simulink model "cl_cm"  (R2021b)
settings: Solver=VariableStepAuto  StartTime=0.0  StopTime=5  RelTol=1e-3
values from neighbouring files (symbols this model uses):
  cl0 = 0.26318895    [model_main.m]
  cla = 5.5497917    [model_main.m]
  clad = 0.008081279    [model_main.m]
  cm0 = 0.08960583    [model_main.m]
  cma = -0.26464918    [model_main.m]
  cmad = -0.018147167    [model_main.m]
  U = 40.00    (= 40)    [model_main.m]
settings Model: Creator=stevenfang  LastModifiedBy=stevenfang

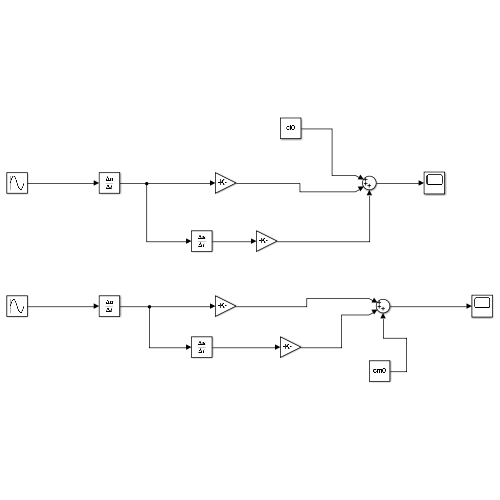
[thumbnail: Simulink's stored preview of the top-level diagram]
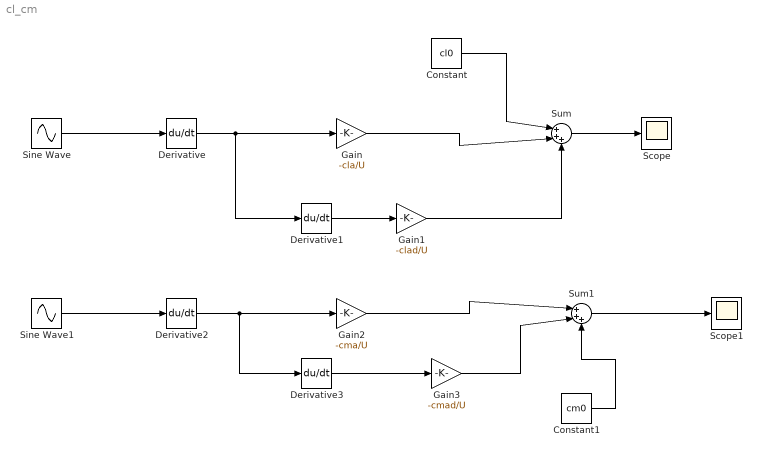
== system cl_cm ==
  Constant : Constant  Value=cl0
  Constant1 : Constant  Value=cm0
  Derivative{,1..3} (4 alike) : Derivative
  Gain : Gain  Gain=-cla/U
  Gain1 : Gain  Gain=-clad/U
  Gain2 : Gain  Gain=-cma/U
  Gain3 : Gain  Gain=-cmad/U
  Scope : Scope
  Scope1 : Scope
  Sine Wave : Sin  Amplitude=0.01  Frequency=5*(2*pi)  SampleTime=0
  Sine Wave1 : Sin  Amplitude=1*(pi/180)  Frequency=5*(2*pi)  SampleTime=0
  Sum : Sum  Inputs=|+++
  Sum1 : Sum  Inputs=|+++
  wires:
  Sine Wave/1 -> Derivative/1
  Derivative/1 -> Derivative1/1, Gain/1
  Derivative1/1 -> Gain1/1
  Sum/1 -> Scope/1
  Gain1/1 -> Sum/3
  Gain/1 -> Sum/2
  Constant/1 -> Sum/1
  Sine Wave1/1 -> Derivative2/1
  Derivative2/1 -> Gain2/1, Derivative3/1
  Derivative3/1 -> Gain3/1
  Gain2/1 -> Sum1/1
  Gain3/1 -> Sum1/2
  Constant1/1 -> Sum1/3
  Sum1/1 -> Scope1/1
